simulink model "c2838xd_ipc_cpu2"  (R2021b)
settings: Solver=FixedStepDiscrete  StartTime=0.0  StopTime=Inf  RelTol=1e-3  EnableMultiTasking=on
undefined symbols (not defined in the file or in its folder): C28x, CPU1, CPU2
libraries: c2837xDlib x8, demo_controls x1
settings Model: ExtModeTrigDuration=8  Creator=The MathWorks, Inc.  LastModifiedBy=The MathWorks, Inc.
settings SolverCC: AlgebraicLoopSolver=TrustRegion  MinimalZcImpactIntegration=on
settings DataIOCC: ReturnWorkspaceOutputs=off
settings OptimizationCC: DefaultUnderspecifiedDataType=single  EnhancedBackFolding=on  StrengthReduction=on  PassReuseOutputArgsAs=Individual arguments  MaxStackSize=1024  OptimizeBlockOrder=speed  DifferentSizesBufferReuse=on  DenormalBehavior=FlushToZero  EfficientTunableParamExpr=on
settings DebuggingCC: ParameterPrecisionLossMsg=none  ParameterTunabilityLossMsg=error  SFMachineParentedDataDiag=warning  ArithmeticOperatorsInVariantConditions=warning
settings HardwareCC: ProdBitPerChar=16  ProdBitPerInt=16  ProdBitPerPointer=32  ProdBitPerSizeT=32  ProdBitPerPtrDiffT=32  ProdLargestAtomicInteger=Integer  ProdLargestAtomicFloat=None  ProdWordSize=16  ProdLongLongMode=on  ProdHWDeviceType=Texas Instruments->C2000
settings SFSimCC: SimUseLocalCustomCode=off  MATLABDynamicMemAlloc=off  CustomCodeUndefinedFunction=UseInterfaceOnly
settings RTWCC: Description=Embedded Coder  SystemTargetFile=ert.tlc  HardwareBoard=TI F2838x (C28x)  TemplateMakefile=ert_default_tmf  GenerateReport=on  RTWUseLocalCustomCode=off  Toolchain=Texas Instruments Code Composer Studio - EABI (C2000)  BuildConfiguration=Debug  IncludeHyperlinkInReport=on  LaunchReport=on  GenerateTraceInfo=on  GenerateTraceReport=on  GenerateTraceReportSl=on  GenerateTraceReportSf=on  GenerateTraceReportEml=on
settings CodeAppCC: ForceParamTrailComments=on  IgnoreCustomStorageClasses=off  OperatorAnnotations=on  SimulinkDataObjDesc=on  SFDataObjDesc=on  InsertBlockDesc=on
settings ERTTargetCC: CodeReplacementLibrary=TI C28x  ExtModeTransport=4  ExtModeStaticAlloc=on  ExtModeStaticAllocSize=10000  ExtModeMexFile=ext_xcp  ExtModeIntrfLevel=Level2 - Open

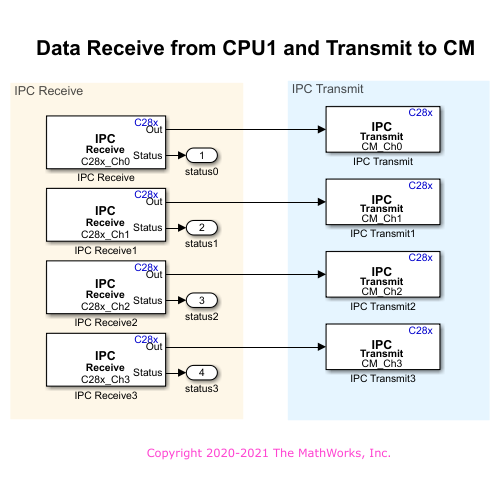
[thumbnail: Simulink's stored preview of the top-level diagram]
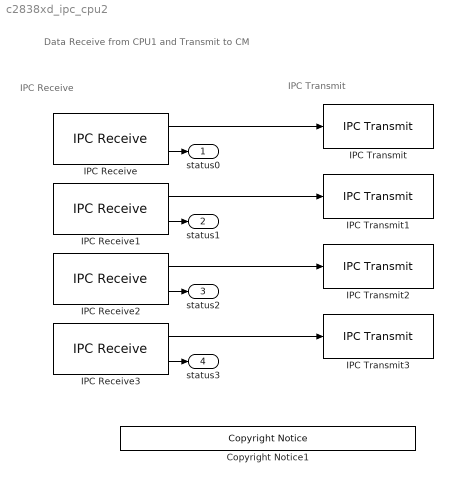
== system c2838xd_ipc_cpu2 ==
  note: IPC Transmit
  note: IPC Receive
  note: Data Receive from CPU1 and Transmit to CM
  Copyright Notice1 : demo_controls/Copyright Notice  year=2020  prod=tic2000
      settings: SourceProductBaseCode=ME
  IPC Receive : c2837xDlib/IPC Receive  blkParamProc=F2838x  SelectSource=C28x (CPU1/CPU2)  SelectChannel=0  DataType=uint16  DataLength=1  EnableBlocking=off  SampleTime=0.25
      settings: SourceProductBaseCode=TIC2000
  IPC Receive1 : c2837xDlib/IPC Receive  blkParamProc=F2838x  SelectSource=C28x (CPU1/CPU2)  SelectChannel=1  DataType=uint16  DataLength=1  EnableBlocking=off  SampleTime=0.5
      settings: SourceProductBaseCode=TIC2000
  IPC Receive2 : c2837xDlib/IPC Receive  blkParamProc=F2838x  SelectSource=C28x (CPU1/CPU2)  SelectChannel=2  DataType=uint16  DataLength=1  EnableBlocking=off  SampleTime=1
      settings: SourceProductBaseCode=TIC2000
  IPC Receive3 : c2837xDlib/IPC Receive  blkParamProc=F2838x  SelectSource=C28x (CPU1/CPU2)  SelectChannel=3  DataType=uint16  DataLength=1  EnableBlocking=off  SampleTime=2
      settings: SourceProductBaseCode=TIC2000
  IPC Transmit : c2837xDlib/IPC Transmit  blkParamProc=F2838x  SelectDestination=ARM Cortex-M4 (CM)  SelectChannel=0  EnableBlocking=off
      settings: SourceProductBaseCode=TIC2000
  IPC Transmit1 : c2837xDlib/IPC Transmit  blkParamProc=F2838x  SelectDestination=ARM Cortex-M4 (CM)  SelectChannel=1  EnableBlocking=off
      settings: SourceProductBaseCode=TIC2000
  IPC Transmit2 : c2837xDlib/IPC Transmit  blkParamProc=F2838x  SelectDestination=ARM Cortex-M4 (CM)  SelectChannel=2  EnableBlocking=off
      settings: SourceProductBaseCode=TIC2000
  IPC Transmit3 : c2837xDlib/IPC Transmit  blkParamProc=F2838x  SelectDestination=ARM Cortex-M4 (CM)  SelectChannel=3  EnableBlocking=off
      settings: SourceProductBaseCode=TIC2000
  status0 : Outport
  status1 : Outport  Port=2
  status2 : Outport  Port=3
  status3 : Outport  Port=4
  wires:
  IPC Receive1/1 -> IPC Transmit1/1
  IPC Receive/1 -> IPC Transmit/1
  IPC Receive3/1 -> IPC Transmit3/1
  IPC Receive/2 -> status0/1
  IPC Receive1/2 -> status1/1
  IPC Receive2/2 -> status2/1
  IPC Receive3/2 -> status3/1
  IPC Receive2/1 -> IPC Transmit2/1
